simulink model "quadrotor_dynamics"  (R2024a)
settings: Solver=VariableStepAuto  StartTime=0.0  StopTime=50  RelTol=1e-3
undefined symbols (not defined in the file): Cm_r, Ct_r, d, g, I_xx, I_yy, I_zz, m, p, phi, psi, q, r, theta, v, w, w_hover, x, y, z
libraries: aerolibobsolete x1, aerolibasang x1
settings Model: Creator=nikhi  LastModifiedBy=nikhi
settings DataIOCC: ExternalInput=getinputstruct(op_trim1)  InitialState=getstatestruct(op_trim1)

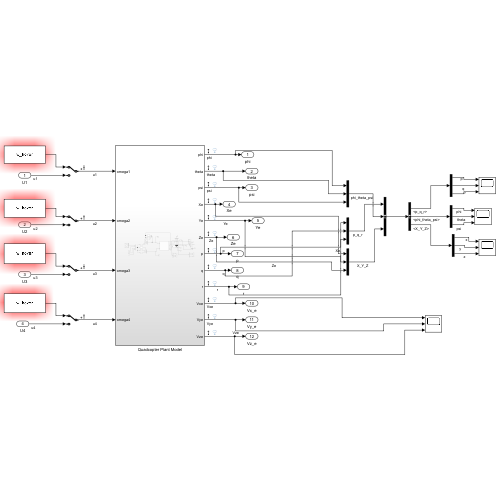
[thumbnail: Simulink's stored preview of the top-level diagram]
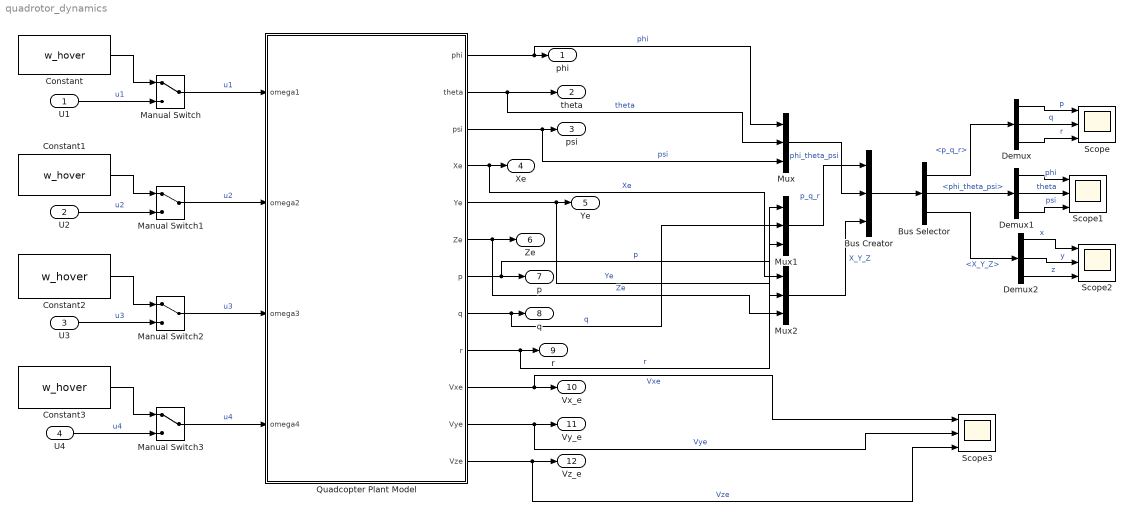
== system quadrotor_dynamics ==
  U1 : Inport
  U2 : Inport  Port=2
  U3 : Inport  Port=3
  U4 : Inport  Port=4
  Bus Creator : BusCreator  Inputs=3
  Bus Selector : BusSelector  OutputSignals=p_q_r,phi_theta_psi,X_Y_Z
  Constant{,1..3} (4 alike) : Constant  Value=w_hover
  Demux : Demux  Outputs=3
  Demux1 : Demux  Outputs=3
  Demux2 : Demux  Outputs=3
  Manual Switch{,1..3} (4 alike) : ManualSwitch
  Mux : Mux  Inputs=3
  Mux1 : Mux  Inputs=3
  Mux2 : Mux  Inputs=3
  Quadcopter Plant Model : Subsystem
  Scope{,1..3} (4 alike) : Scope  NumInputPorts=3
  phi : Outport
  theta : Outport  Port=2
  psi : Outport  Port=3
  Xe : Outport  Port=4
  Ye : Outport  Port=5
  Ze : Outport  Port=6
  p : Outport  Port=7
  q : Outport  Port=8
  r : Outport  Port=9
  Vx_e : Outport  Port=10
  Vy_e : Outport  Port=11
  Vz_e : Outport  Port=12
  wires:
  Quadcopter Plant Model/2(theta) -> Mux/2, theta/1  "theta"
  Quadcopter Plant Model/7(p) -> Mux1/1, p/1  "p"
  Quadcopter Plant Model/10(Vxe) -> Scope3/1, Vx_e/1  "Vxe"
  Quadcopter Plant Model/4(Xe) -> Xe/1, Mux2/1  "Xe"
  Quadcopter Plant Model/9(r) -> r/1, Mux1/3  "r"
  Quadcopter Plant Model/8(q) -> Mux1/2, q/1  "q"
  Quadcopter Plant Model/1(phi) -> Mux/1, phi/1  "phi"
  Quadcopter Plant Model/5(Ye) -> Mux2/2, Ye/1  "Ye"
  Quadcopter Plant Model/3(psi) -> Mux/3, psi/1  "psi"
  Quadcopter Plant Model/11(Vye) -> Scope3/2, Vy_e/1  "Vye"
  Quadcopter Plant Model/12(Vze) -> Scope3/3, Vz_e/1  "Vze"
  Quadcopter Plant Model/6(Ze) -> Mux2/3, Ze/1  "Ze"
  Mux1/1 -> Bus Creator/1  "p_q_r"
  Mux/1 -> Bus Creator/2  "phi_theta_psi"
  Mux2/1 -> Bus Creator/3  "X_Y_Z"
  Bus Creator/1 -> Bus Selector/1
  Bus Selector/2 -> Demux1/1  "<phi_theta_psi>"
  Bus Selector/1 -> Demux/1  "<p_q_r>"
  Bus Selector/3 -> Demux2/1  "<X_Y_Z>"
  Demux/2 -> Scope/2  "q"
  Demux/1 -> Scope/1  "p"
  Demux/3 -> Scope/3  "r"
  Demux1/2 -> Scope1/2  "theta"
  Demux1/1 -> Scope1/1  "phi"
  Demux1/3 -> Scope1/3  "psi"
  Demux2/1 -> Scope2/1  "x"
  Demux2/2 -> Scope2/2  "y"
  Demux2/3 -> Scope2/3  "z"
  U1/1 -> Manual Switch/2  "u1"
  Manual Switch/1 -> Quadcopter Plant Model/1(omega1)  "u1"
  Constant/1 -> Manual Switch/1
  Manual Switch1/1 -> Quadcopter Plant Model/2(omega2)  "u2"
  U2/1 -> Manual Switch1/2  "u2"
  U4/1 -> Manual Switch3/2  "u4"
  U3/1 -> Manual Switch2/2  "u3"
  Manual Switch2/1 -> Quadcopter Plant Model/3(omega3)  "u3"
  Manual Switch3/1 -> Quadcopter Plant Model/4(omega4)  "u4"
  Constant1/1 -> Manual Switch1/1
  Constant2/1 -> Manual Switch2/1
  Constant3/1 -> Manual Switch3/1

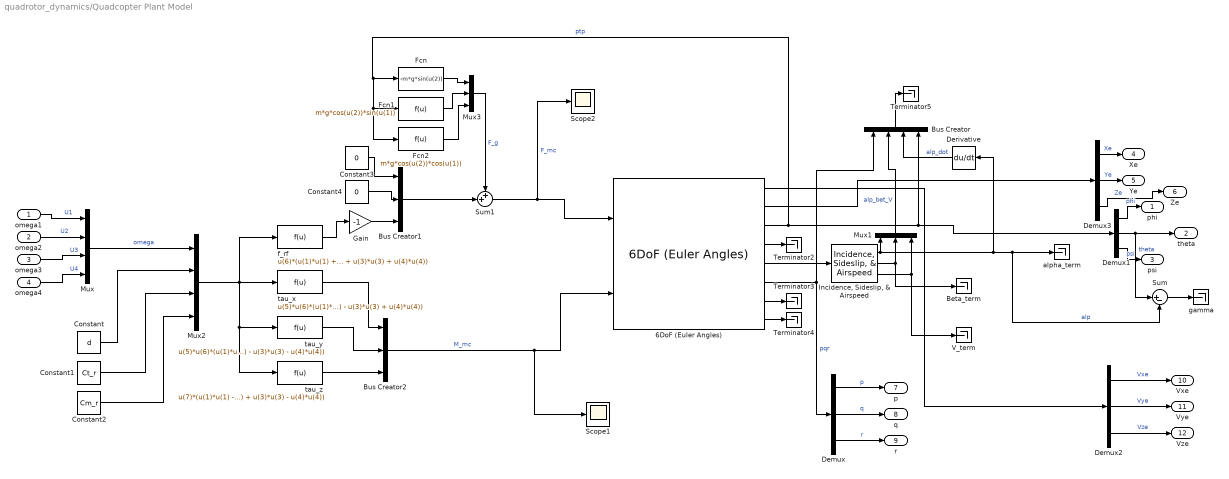
== system quadrotor_dynamics/Quadcopter Plant Model ==
  omega1 : Inport
  omega2 : Inport  Port=2
  omega3 : Inport  Port=3
  omega4 : Inport  Port=4
  6DoF (Euler Angles) : aerolibobsolete/6DoF (Euler Angles)  units=Metric (MKS)  mtype=Fixed  rep=Euler Angles  xme_0=[x y z]  Vm_0=[u v w]  eul_0=[phi theta psi]  pm_0=[p q r]  mass_0=m  mass_e=0.5  mass_f=2.0  inertia=diag([I_xx I_yy I_zz])  inertia_e=eye(3)  inertia_f=2*eye(3)  k_quat=1.0
  Beta_term : Terminator
  Bus Creator : BusCreator  Inputs=4
  Bus Creator1 : BusCreator  Inputs=3
  Bus Creator2 : BusCreator  Inputs=3
  Constant : Constant  Value=d
  Constant1 : Constant  Value=Ct_r
  Constant2 : Constant  Value=Cm_r
  Constant3 : Constant  Value=0
  Constant4 : Constant  Value=0
  Demux{,1..3} (4 alike) : Demux  Outputs=3
  Derivative : Derivative
  Fcn : Fcn  Expr=-m*g*sin(u(2))
  Fcn1 : Fcn  Expr=m*g*cos(u(2))*sin(u(1))
  Fcn2 : Fcn  Expr=m*g*cos(u(2))*cos(u(1))
  Gain : Gain  Gain=-1
  "Incidence, Sideslip, & Airspeed" : aerolibasang/Incidence, Sideslip, & Airspeed
  Mux : Mux
  Mux1 : Mux  Inputs=3
  Mux2 : Mux
  Mux3 : Mux  Inputs=3
  Scope1 : Scope
  Scope2 : Scope
  Sum : Sum  Inputs=|+-
  Sum1 : Sum  Inputs=++|
  Terminator{2..5} (4 alike) : Terminator
  V_term : Terminator
  alpha_term : Terminator
  f_rf : Fcn  Expr=u(6)*(u(1)*u(1) + u(2)*u(2) + u(3)*u(3) + u(4)*u(4))
  gamma : Terminator
  tau_x : Fcn  Expr=u(5)*u(6)*(u(1)*u(1) - u(2)*u(2) - u(3)*u(3) + u(4)*u(4))
  tau_y : Fcn  Expr=u(5)*u(6)*(u(1)*u(1) + u(2)*u(2) - u(3)*u(3) - u(4)*u(4))
  tau_z : Fcn  Expr=u(7)*(u(1)*u(1) - u(2)*u(2) + u(3)*u(3) - u(4)*u(4))
  phi : Outport
  theta : Outport  Port=2
  psi : Outport  Port=3
  Xe : Outport  Port=4
  Ye : Outport  Port=5
  Ze : Outport  Port=6
  p : Outport  Port=7
  q : Outport  Port=8
  r : Outport  Port=9
  Vxe : Outport  Port=10
  Vye : Outport  Port=11
  Vze : Outport  Port=12
  wires:
  Demux/2 -> q/1  "q"
  Demux1/2 -> theta/1, Sum/1  "theta"
  "Incidence, Sideslip, & Airspeed"/3 -> V_term/1, Mux1/3
  Demux3/3 -> Ze/1  "Ze"
  6DoF (Euler Angles)/6 -> Bus Creator/1, Demux/1  "pqr"
  Derivative/1 -> Bus Creator/3  "alp_dot"
  6DoF (Euler Angles)/7 -> Terminator3/1
  "Incidence, Sideslip, & Airspeed"/1 -> alpha_term/1, Sum/2, Derivative/1, Mux1/1  "alp"
  "Incidence, Sideslip, & Airspeed"/2 -> Beta_term/1, Mux1/2
  6DoF (Euler Angles)/2 -> Demux3/1
  Mux1/1 -> Bus Creator/2  "alp_bet_V"
  Demux1/3 -> psi/1  "psi"
  6DoF (Euler Angles)/3 -> Fcn2/1, Fcn1/1, Fcn/1, Bus Creator/4, Demux1/1  "ptp"
  Demux1/1 -> phi/1  "phi"
  6DoF (Euler Angles)/8 -> Terminator4/1
  Demux3/2 -> Ye/1  "Ye"
  Demux/3 -> r/1  "r"
  6DoF (Euler Angles)/4 -> Terminator2/1
  6DoF (Euler Angles)/5 -> "Incidence, Sideslip, & Airspeed"/1
  Demux3/1 -> Xe/1  "Xe"
  Demux/1 -> p/1  "p"
  6DoF (Euler Angles)/1 -> Demux2/1
  Demux2/1 -> Vxe/1  "Vxe"
  Demux2/2 -> Vye/1  "Vye"
  Demux2/3 -> Vze/1  "Vze"
  Bus Creator/1 -> Terminator5/1
  omega1/1 -> Mux/1  "U1"
  omega2/1 -> Mux/2  "U2"
  omega3/1 -> Mux/3  "U3"
  omega4/1 -> Mux/4  "U4"
  Mux/1 -> Mux2/1  "omega"
  Sum/1 -> gamma/1
  Constant1/1 -> Mux2/3
  Constant/1 -> Mux2/2
  Constant2/1 -> Mux2/4
  Mux2/1 -> tau_z/1, tau_y/1, tau_x/1, f_rf/1
  Constant4/1 -> Bus Creator1/2
  f_rf/1 -> Gain/1
  Sum1/1 -> Scope2/1, 6DoF (Euler Angles)/1  "F_mc"
  Bus Creator2/1 -> Scope1/1, 6DoF (Euler Angles)/2  "M_mc"
  Constant3/1 -> Bus Creator1/1
  Gain/1 -> Bus Creator1/3
  tau_y/1 -> Bus Creator2/2
  tau_z/1 -> Bus Creator2/3
  tau_x/1 -> Bus Creator2/1
  Bus Creator1/1 -> Sum1/2
  Fcn/1 -> Mux3/1
  Fcn1/1 -> Mux3/2
  Fcn2/1 -> Mux3/3
  Mux3/1 -> Sum1/1  "F_g"
